simulink model "sim_pos_dist_obs_tcas"  (R2020a)
settings: Solver=ode4  StartTime=0.0  StopTime=30.0  FixedStep=0.01  RelTol=1e-3
values from neighbouring files (symbols this model uses):
  alfa_theta = 20    [draw_compare_dist_pos_obs.m]
  alfa_theta_obs = 100    [draw_compare_dist_pos_obs.m]
  beta1 = 1.2    [draw_compare_dist_pos_obs.m]
  beta2 = 0.8    [draw_compare_dist_pos_obs.m]
  delta_p_i_0 = zeros(3, NF)    [draw_compare_dist_pos_obs.m]
  delta_v_i_0 = zeros(3, NF)    [draw_compare_dist_pos_obs.m]
  dp_aa_t = 0.2 * ones(3, 5) + ( 1.0 - 0.2 ) * rand(3, 5)    [draw_compare_dist_pos_obs.m]
  dp_ff_t = [ 0.4 * ones(1, 5) + ( 1.0 - 0.4 ) * rand(1, 5);                      0.4 * ones(1, 5) + ( 1.0 - 0.4 ) * rand(1, 5);                      0.2 * ones(1, 5) + ( 0.6 - 0.2 ) * rand(1, 5) ]    [draw_compare_dist_pos_obs.m]
  dp_phi_t = ( - pi / 2 ) * ones(3, 5) + ( pi / 2 - ( - pi / 2 ) ) * rand(3, 5)    [draw_compare_dist_pos_obs.m]
  ell1 = [100; 100; 100]    [draw_compare_dist_pos_obs.m]
  ell2 = [50; 50; 50]    [draw_compare_dist_pos_obs.m]
  ell3 = [5; 5; 5]    [draw_compare_dist_pos_obs.m]
  epv = [0.1; 0.1; 0.1]    [draw_compare_dist_pos_obs.m]
  etai_0 = zeros(3,5)    [draw_compare_dist_pos_obs.m]
  k0 = [10; 10; 10]    [draw_compare_dist_pos_obs.m]
  k1v = [0.1; 0.1; 0.1]    [draw_compare_dist_pos_obs.m]
  k2v = [0.1; 0.1; 0.1]    [draw_compare_dist_pos_obs.m]
  k3v = [0.01; 0.01; 0.01]    [draw_compare_dist_pos_obs.m]
  kai_1_t = 0.02    [draw_compare_dist_pos_obs.m]
  kai_3_t = 0.1    [draw_compare_dist_pos_obs.m]
  kai_chi_1 = diag([6; 6; 6])    [draw_compare_dist_pos_obs.m]
  kai_chi_2 = diag([6; 6; 6])    [draw_compare_dist_pos_obs.m]
  kai_u_1 = diag([8; 8; 8])    [draw_compare_dist_pos_obs.m]
  kai_u_2 = diag([8; 8; 8])    [draw_compare_dist_pos_obs.m]
  ksii_0 = zeros(3,5)    [draw_compare_dist_pos_obs.m]
  l1v = diag([20; 20; 20])    [draw_compare_dist_pos_obs.m]
  l2v = diag([30; 30; 30])    [draw_compare_dist_pos_obs.m]
  mass_i = zeros(1,NF)    [draw_compare_dist_pos_obs.m]
  Mii = diag([1;0;0;0;1])    [draw_compare_dist_pos_obs.m]
  pos0 = zeros(3, 1)    [draw_compare_dist_pos_obs.m]
  PZ0 = P0(3)    [draw_compare_dist_pos_obs.m]
  PZ1 = 10    [draw_compare_dist_pos_obs.m]
  Qci_init = repmat([1;0;0;0],1,NF)    [draw_compare_dist_pos_obs.m]
  R0 = 4    [draw_compare_dist_pos_obs.m]
  R1 = 8    [draw_compare_dist_pos_obs.m]
  Rx2 = 10    [draw_compare_dist_pos_obs.m]
  Ry2 = 6    [draw_compare_dist_pos_obs.m]
  Rz2 = 4    [draw_compare_dist_pos_obs.m]
  T0 = 0    [draw_compare_dist_pos_obs.m]
  T1 = tseq1    (= 10)    [draw_compare_dist_pos_obs.m]
  T12 = tseq1 + tseq12    (= 20)    [draw_compare_dist_pos_obs.m]
  T2 = tseq1 + tseq12 + tseq2    (= 30)    [draw_compare_dist_pos_obs.m]
  theta0 = ( 2 / 5 ) * pi    (= 1.25663706144)    [draw_compare_dist_pos_obs.m]
  vel0 = zeros(3, 1)    [draw_compare_dist_pos_obs.m]
  Wij = [0,0,1,0,0;              0,0,1,1,0;              1,0,0,0,1;              0,1,1,0,0;              0,0,1,0,0]    [draw_compare_dist_pos_obs.m]
  X1 = 8    [draw_compare_dist_pos_obs.m]
  X2 = 2    [draw_compare_dist_pos_obs.m]
  X3 = 3    [draw_compare_dist_pos_obs.m]
  Y1 = 10    [draw_compare_dist_pos_obs.m]
  Y2 = 2    [draw_compare_dist_pos_obs.m]
  Y3 = 4    [draw_compare_dist_pos_obs.m]
  Z1 = 4    [draw_compare_dist_pos_obs.m]
  Z2 = -6    [draw_compare_dist_pos_obs.m]
  Z3 = 2    [draw_compare_dist_pos_obs.m]
undefined symbols (not defined in the file or in its folder): cal_frac_squ, p_alfa_1, p_alfa_2, p_beta1, p_beta2, p_dbeta1, p_dbeta2, p_gamma1_pos, p_gamma1_vel, p_gamma2_pos, p_gamma2_vel, q_alfa_1, q_alfa_2, q_beta1, q_beta2, q_dbeta1, q_dbeta2, q_gamma1_pos, q_gamma1_vel, q_gamma2_pos, q_gamma2_vel
(part 2 of 4)

== matlab function sim_pos_dist_obs_tcas/choose ksi_est_err 19 ==
  data: x input; y output
function y = fcn(x)
iiuav = 5;
y = x(:,iiuav);

== matlab function sim_pos_dist_obs_tcas/leader control input ==
  data: t input; u0 output; T1 input; T2 input; R0 input; R1 input; Rx2 input; Ry2 input; Rz2 input
function u0  = fcn(t, T1, T2, R0, R1, Rx2, Ry2, Rz2)
%%%% 给出领导者参考加速度控制输入
u0 = zeros(3, 1);

if t <= ( T1 + 1e-05 )
    u0(1, 1) = - ( 4 * pi * sin( ( 2 * pi * ( t - 0 ) ) / ( 0 - T1 ) ) * ( R0 - R1 ) ) / ( ( 0 - T1 ) ^ 2 ) ...
                        - ( 4 * ( pi ^ 2 ) * cos( ( 2 * pi * ( t - 0 ) ) / ( 0 - T1 ) ) ...
                        * ( R0 + ( ( R0 - R1 ) * ( t - 0 ) ) / ( 0 - T1 ) ) ) / ( ( 0 - T1 ) ^ 2 );
    u0(2, 1) = ( 4 * pi * cos( ( 2 * pi * ( t - 0 ) ) / ( 0 - T1 ) ) * ( R0 - R1 ) ) / ( ( 0 - T1 ) ^ 2 ) ...
                        - ( 4 * ( pi ^ 2 ) * sin( ( 2 * pi * ( t - 0 ) ) / ( 0 - T1 ) ) ...
                        * ( R0 + ( ( R0 - R1 ) * ( t - 0 ) ) / ( 0 - T1 ) ) ) / ( ( 0 - T1 ) ^ 2 );
    u0(3, 1) = 0;
else
    u0(1, 1) = ( 4 * Rx2 * ( pi ^ 2 ) * cos( ( 2 * pi * ( t - T1 ) ) / ( T1 - T2 ) ) ) / ( ( T1 - T2 ) ^ 2 );
    u0(2, 1) = - ( 16 * Ry2 * ( pi ^ 2 ) * sin( ( 4 * pi * ( t - T1 ) ) / ( T1 - T2 ) ) ) / ( ( T1 - T2 ) ^ 2 );
    u0(3, 1) = ( 16 * Rz2 * ( pi ^ 2 ) * sin( ( 4 * pi * ( t - T1 ) ) / ( T1 - T2 ) ) ) / ( ( T1 - T2 ) ^ 2 );
end

== matlab function sim_pos_dist_obs_tcas/choose ksi_est_err 20 ==
  data: x input; y output
function y = fcn(x)
iiuav = 5;
y = x(:,iiuav);

== matlab function sim_pos_dist_obs_tcas/trans to column18 ==
  data: x input; y output
function y = fcn(x)
y = x(:);

== matlab function sim_pos_dist_obs_tcas/trans to column19 ==
  data: x input; y output
function y = fcn(x)
y = x(:);

== matlab function sim_pos_dist_obs_tcas/cal dchi agent 1 ==
  data: kai_chi_1 input; d_chi_1 output; kai_chi_2 input; d_theta_err_ksi_1_vec input; d_theta_err_ksi_2_vec input
function d_chi_1 = fcn(kai_chi_1, kai_chi_2, d_theta_err_ksi_1_vec, d_theta_err_ksi_2_vec)
%%%% 固定时间虚拟速度控制量导数d_chi
iiuav = 1;
d_chi_1 = -kai_chi_1 * d_theta_err_ksi_1_vec(:,iiuav) - kai_chi_2 * d_theta_err_ksi_2_vec(:,iiuav);

== matlab function sim_pos_dist_obs_tcas/combine dtheta_err_ksi ==
  data: d_theta_err_ksi_1_1 input; d_theta_err_ksi_1_2 input; d_theta_err_ksi_1_3 input; d_theta_err_ksi_1_4 input; d_theta_err_ksi_1_5 input; d_theta_err_ksi_1_vec output; d_theta_err_ksi_2_1 input; d_theta_err_ksi_2_vec output; d_theta_err_ksi_2_2 input; d_theta_err_ksi_2_3 input; d_theta_err_ksi_2_4 input; d_theta_err_ksi_2_5 input
function [d_theta_err_ksi_1_vec, d_theta_err_ksi_2_vec]  = fcn(d_theta_err_ksi_1_1, d_theta_err_ksi_1_2, d_theta_err_ksi_1_3, d_theta_err_ksi_1_4, d_theta_err_ksi_1_5, ...
                                                                                                                d_theta_err_ksi_2_1, d_theta_err_ksi_2_2, d_theta_err_ksi_2_3, d_theta_err_ksi_2_4, d_theta_err_ksi_2_5)
%%%% 合并平滑函数的导数
d_theta_err_ksi_1_vec = [d_theta_err_ksi_1_1(:), d_theta_err_ksi_1_2(:), d_theta_err_ksi_1_3(:), d_theta_err_ksi_1_4(:), d_theta_err_ksi_1_5(:)];
d_theta_err_ksi_2_vec = [d_theta_err_ksi_2_1(:), d_theta_err_ksi_2_2(:), d_theta_err_ksi_2_3(:), d_theta_err_ksi_2_4(:), d_theta_err_ksi_2_5(:)];

== matlab function sim_pos_dist_obs_tcas/cal dchi agent 2 ==
  data: kai_chi_1 input; d_chi_2 output; kai_chi_2 input; d_theta_err_ksi_1_vec input; d_theta_err_ksi_2_vec input
function d_chi_2 = fcn(kai_chi_1, kai_chi_2, d_theta_err_ksi_1_vec, d_theta_err_ksi_2_vec)
%%%% 固定时间虚拟速度控制量导数d_chi
iiuav = 2;
d_chi_2 = -kai_chi_1 * d_theta_err_ksi_1_vec(:,iiuav) - kai_chi_2 * d_theta_err_ksi_2_vec(:,iiuav);

== matlab function sim_pos_dist_obs_tcas/cal dchi agent 3 ==
  data: kai_chi_1 input; d_chi_3 output; kai_chi_2 input; d_theta_err_ksi_1_vec input; d_theta_err_ksi_2_vec input
function d_chi_3 = fcn(kai_chi_1, kai_chi_2, d_theta_err_ksi_1_vec, d_theta_err_ksi_2_vec)
%%%% 固定时间虚拟速度控制量导数d_chi
iiuav = 3;
d_chi_3 = -kai_chi_1 * d_theta_err_ksi_1_vec(:,iiuav) - kai_chi_2 * d_theta_err_ksi_2_vec(:,iiuav);

== matlab function sim_pos_dist_obs_tcas/cal dchi agent 4 ==
  data: kai_chi_1 input; d_chi_4 output; kai_chi_2 input; d_theta_err_ksi_1_vec input; d_theta_err_ksi_2_vec input
function d_chi_4 = fcn(kai_chi_1, kai_chi_2, d_theta_err_ksi_1_vec, d_theta_err_ksi_2_vec)
%%%% 固定时间虚拟速度控制量导数d_chi
iiuav = 4;
d_chi_4 = -kai_chi_1 * d_theta_err_ksi_1_vec(:,iiuav) - kai_chi_2 * d_theta_err_ksi_2_vec(:,iiuav);

== matlab function sim_pos_dist_obs_tcas/cal dchi agent 5 ==
  data: kai_chi_1 input; d_chi_5 output; kai_chi_2 input; d_theta_err_ksi_1_vec input; d_theta_err_ksi_2_vec input
function d_chi_5 = fcn(kai_chi_1, kai_chi_2, d_theta_err_ksi_1_vec, d_theta_err_ksi_2_vec)
%%%% 固定时间虚拟速度控制量导数d_chi
iiuav = 5;
d_chi_5 = -kai_chi_1 * d_theta_err_ksi_1_vec(:,iiuav) - kai_chi_2 * d_theta_err_ksi_2_vec(:,iiuav);

== matlab function sim_pos_dist_obs_tcas/combine dchi ==
  data: d_chi_1 input; d_chi_2 input; d_chi_3 input; d_chi_4 input; d_chi_5 input; d_chi_vec output
function d_chi_vec  = fcn(d_chi_1, d_chi_2, d_chi_3, d_chi_4, d_chi_5)
%%%% 合并领导者位置观测器输出结果
d_chi_vec = [d_chi_1(:), d_chi_2(:), d_chi_3(:), d_chi_4(:), d_chi_5(:)];

== matlab function sim_pos_dist_obs_tcas/cal abs 22 ==
  data: x input; y output
function y = fcn(x)
y = abs(x(:));

== matlab function sim_pos_dist_obs_tcas/choose ksi_est_err 21 ==
  data: x input; y output
function y = fcn(x)
iiuav = 1;
y = x(:,iiuav);

== matlab function sim_pos_dist_obs_tcas/cal x1_tilt ==
  data: ksi_i_vec input; x1_hat_vec input; x1_tilt_vec output
function x1_tilt_vec = fcn(ksi_i_vec, x1_hat_vec)
%%%% 计算状态观测误差
x1_tilt_vec = zeros(3,5);
for iiuav = 1:5
    x1_tilt_vec(:,iiuav) = ksi_i_vec(:,iiuav) - x1_hat_vec(:,iiuav);
end

== matlab function sim_pos_dist_obs_tcas/cal err_1_x1_tilt ==
  data: ell1 input; epv input; err_1_x1_tilt_vec output; x1_tilt_vec input
function err_1_x1_tilt_vec = fcn(ell1, epv, x1_tilt_vec)
%%%% 计算状态观测误差
err_1_x1_tilt_vec = zeros(3,5);
for iiuav = 1:5
    err_1_x1_tilt_vec(:,iiuav) = (1 ./ (ell1(:) .* (epv(:) .^ 2))) .* x1_tilt_vec(:,iiuav);
end

== matlab function sim_pos_dist_obs_tcas/cal err_2_x1_tilt ==
  data: ell2 input; epv input; err_2_x1_tilt_vec output; x1_tilt_vec input
function err_2_x1_tilt_vec = fcn(ell2, epv, x1_tilt_vec)
%%%% 计算状态观测误差
err_2_x1_tilt_vec = zeros(3,5);
for iiuav = 1:5
    err_2_x1_tilt_vec(:,iiuav) = (1 ./ (ell2(:) .* (epv(:) .^ 2))) .* x1_tilt_vec(:,iiuav);
end

== matlab function sim_pos_dist_obs_tcas/generate translational disturbance agent 5 ==
  data: dp_aa_t input; dp_ff_t input; dp_phi_t input; dp_5 output; t input
function dp_5 = fcn(dp_aa_t, dp_ff_t, dp_phi_t, t)
%%%% 平移动力学方程中的扰动项设置
epsil_t = zeros(3, 1);

for kk = 1:5
    epsil_t = epsil_t + dp_aa_t(:, kk) .* sin( 2 * pi * dp_ff_t(:, kk) * t + dp_phi_t(:, kk) );
end

dp_5 = [ epsil_t(1) + 1.6 * sin( 0.2 * t ) + 2.0 * cos( 0.3 * t ) + 1.4 * sin( 0.5 * t ) ...
                + 4 * exp( -0.1 * t ) * sin( 0.5 * t ) + 3 / ( 1 + exp( -0.2 * ( t - 15 ) ) ); ...
                epsil_t(2) + 1.2 * sin( 0.1 * t ) + 3 * cos( 0.2 * t ) + 0.8 * sin( 0.4 * t ) ...
                + 2 * exp( -0.15 * t ) * cos( 0.6 * t ) + 3 / ( 1 + exp( -0.3 * ( t - 25 ) ) ); ...
                epsil_t(3) + 1.8 * sin( 0.1 * t ) + 1.6 * sin( 0.2 * t ) + 1.6 * cos( 0.3 * t ) ...
                + 4 * exp( -0.05 * t ) * sin( 0.4 * t + pi / 4 ) + 3 / ( 1 + exp( -0.5 * ( t - 20 ) ) ) ];

== matlab function sim_pos_dist_obs_tcas/cal err_3_x1_tilt ==
  data: ell3 input; epv input; err_3_x1_tilt_vec output; x1_tilt_vec input
function err_3_x1_tilt_vec = fcn(ell3, epv, x1_tilt_vec)
%%%% 计算状态观测误差
err_3_x1_tilt_vec = zeros(3,5);
for iiuav = 1:5
    err_3_x1_tilt_vec(:,iiuav) = (ell3(:) ./ (epv(:) .^ 2)) .* x1_tilt_vec(:,iiuav);
end

== matlab function sim_pos_dist_obs_tcas/cal abs 23 ==
  data: x input; y output
function y = fcn(x)
y = abs(x(:));

== matlab function sim_pos_dist_obs_tcas/cal abs 24 ==
  data: x input; y output
function y = fcn(x)
y = abs(x(:));

== matlab function sim_pos_dist_obs_tcas/choose ksi_est_err 22 ==
  data: x input; y output
function y = fcn(x)
iiuav = 1;
y = x(:,iiuav);

== matlab function sim_pos_dist_obs_tcas/choose ksi_est_err 23 ==
  data: x input; y output
function y = fcn(x)
iiuav = 1;
y = x(:,iiuav);

== matlab function sim_pos_dist_obs_tcas/choose ksi_est_err 24 ==
  data: x input; y output
function y = fcn(x)
iiuav = 1;
y = x(:,iiuav);

== matlab function sim_pos_dist_obs_tcas/trans to column20 ==
  data: x input; y output
function y = fcn(x)
y = x(:);

== matlab function sim_pos_dist_obs_tcas/cal abs 25 ==
  data: x input; y output
function y = fcn(x)
y = abs(x(:));

== matlab function sim_pos_dist_obs_tcas/cal abs 26 ==
  data: x input; y output
function y = fcn(x)
y = abs(x(:));

== matlab function sim_pos_dist_obs_tcas/choose ksi_est_err 25 ==
  data: x input; y output
function y = fcn(x)
iiuav = 1;
y = x(:,iiuav);

== matlab function sim_pos_dist_obs_tcas/choose ksi_est_err 26 ==
  data: x input; y output
function y = fcn(x)
iiuav = 1;
y = x(:,iiuav);

== matlab function sim_pos_dist_obs_tcas/trans to column21 ==
  data: x input; y output
function y = fcn(x)
y = x(:);

== matlab function sim_pos_dist_obs_tcas/trans to column22 ==
  data: x input; y output
function y = fcn(x)
y = x(:);

== matlab function sim_pos_dist_obs_tcas/cal G_fun_x1_tilt agent 2 ==
  data: err_1_x1_tilt_vec input; err_2_x1_tilt_vec input; G_fun_x1_tilt_1_2 output; err_3_x1_tilt_vec input; err_x1_alfa_squ_1_2 input; G_fun_x1_tilt_2_2 output; err_x1_alfa_squ_2_2 input; err_x1_alfa_squ_3_2 input; err_x1_alfa_squ_4_2 input; err_x1_alfa_squ_5_2 input; err_x1_alfa_squ_6_2 input; G_fun_x1_tilt_3_2 output
function [G_fun_x1_tilt_1_2, G_fun_x1_tilt_2_2, G_fun_x1_tilt_3_2] = fcn(err_1_x1_tilt_vec, err_2_x1_tilt_vec, err_3_x1_tilt_vec, ...
                                                                                                                                err_x1_alfa_squ_1_2, err_x1_alfa_squ_2_2, err_x1_alfa_squ_3_2, ...
                                                                                                                                err_x1_alfa_squ_4_2, err_x1_alfa_squ_5_2, err_x1_alfa_squ_6_2)
%%%% 计算平滑递增函数
iiuav = 2;
G_fun_x1_tilt_1_2 = tanh(err_x1_alfa_squ_2_2(:)) .* err_x1_alfa_squ_1_2(:) .* sign(err_1_x1_tilt_vec(:,iiuav));
G_fun_x1_tilt_2_2 = tanh(err_x1_alfa_squ_4_2(:)) .* err_x1_alfa_squ_3_2(:) .* sign(err_2_x1_tilt_vec(:,iiuav));
G_fun_x1_tilt_3_2 = tanh(err_x1_alfa_squ_6_2(:)) .* err_x1_alfa_squ_5_2(:) .* sign(err_3_x1_tilt_vec(:,iiuav));

== matlab function sim_pos_dist_obs_tcas/combine translational disturbance ==
  data: dp_vec output; dp_1 input; dp_2 input; dp_3 input; dp_4 input; dp_5 input
function dp_vec = fcn(dp_1, dp_2, dp_3, dp_4, dp_5)
%%%% 合并领导者编队跟踪误差结果
dp_vec = [dp_1(:), dp_2(:), dp_3(:), dp_4(:), dp_5(:)];

== matlab function sim_pos_dist_obs_tcas/cal abs 27 ==
  data: x input; y output
function y = fcn(x)
y = abs(x(:));

== matlab function sim_pos_dist_obs_tcas/cal abs 28 ==
  data: x input; y output
function y = fcn(x)
y = abs(x(:));

== matlab function sim_pos_dist_obs_tcas/cal abs 29 ==
  data: x input; y output
function y = fcn(x)
y = abs(x(:));

== matlab function sim_pos_dist_obs_tcas/cal Rei ==
  data: Rei output; Qei input
function Rei = fcn(Qei)
%%%% 使用罗德里格公式由四元数Qei求解Rei
Rei = zeros(3,3,5);
for iuav = 1:5
    thetaei_tmp = Qei(1,iuav);
    qei_tmp = Qei(2:4,iuav);
    Rei(:,:,iuav) = ((thetaei_tmp^2) - (qei_tmp')*qei_tmp) * eye(3,3) ...
                            + 2 * qei_tmp * (qei_tmp') ...
                            - 2 * thetaei_tmp * cal_askew_mat(qei_tmp);
end

end

== matlab function sim_pos_dist_obs_tcas/cal abs 30 ==
  data: x input; y output
function y = fcn(x)
y = abs(x(:));

== matlab function sim_pos_dist_obs_tcas/cal abs 61 ==
  data: x input; y output
function y = fcn(x)
y = abs(x(:));

== matlab function sim_pos_dist_obs_tcas/cal abs 62 ==
  data: x input; y output
function y = fcn(x)
y = abs(x(:));

== matlab function sim_pos_dist_obs_tcas/choose ksi_est_err 27 ==
  data: x input; y output
function y = fcn(x)
iiuav = 2;
y = x(:,iiuav);

== matlab function sim_pos_dist_obs_tcas/choose ksi_est_err 28 ==
  data: x input; y output
function y = fcn(x)
iiuav = 2;
y = x(:,iiuav);

== matlab function sim_pos_dist_obs_tcas/choose ksi_est_err 29 ==
  data: x input; y output
function y = fcn(x)
iiuav = 2;
y = x(:,iiuav);

== matlab function sim_pos_dist_obs_tcas/choose ksi_est_err 30 ==
  data: x input; y output
function y = fcn(x)
iiuav = 2;
y = x(:,iiuav);

== matlab function sim_pos_dist_obs_tcas/choose ksi_est_err 41 ==
  data: x input; y output
function y = fcn(x)
iiuav = 2;
y = x(:,iiuav);

== matlab function sim_pos_dist_obs_tcas/choose ksi_est_err 42 ==
  data: x input; y output
function y = fcn(x)
iiuav = 2;
y = x(:,iiuav);

== matlab function sim_pos_dist_obs_tcas/trans to column23 ==
  data: x input; y output
function y = fcn(x)
y = x(:);

== matlab function sim_pos_dist_obs_tcas/cal abs 2 ==
  data: x input; y output
function y = fcn(x)
y = abs(x(:));

== matlab function sim_pos_dist_obs_tcas/trans to column24 ==
  data: x input; y output
function y = fcn(x)
y = x(:);

== matlab function sim_pos_dist_obs_tcas/trans to column25 ==
  data: x input; y output
function y = fcn(x)
y = x(:);

== matlab function sim_pos_dist_obs_tcas/trans to column26 ==
  data: x input; y output
function y = fcn(x)
y = x(:);

== matlab function sim_pos_dist_obs_tcas/trans to column27 ==
  data: x input; y output
function y = fcn(x)
y = x(:);

== matlab function sim_pos_dist_obs_tcas/trans to column28 ==
  data: x input; y output
function y = fcn(x)
y = x(:);

== matlab function sim_pos_dist_obs_tcas/depart Re5 ==
  data: y output; x input
function y = fcn(x)
y = x(:,:,5);

end

== matlab function sim_pos_dist_obs_tcas/depart Re1 ==
  data: y output; x input
function y = fcn(x)
y = x(:,:,1);

end

== matlab function sim_pos_dist_obs_tcas/depart Re2 ==
  data: y output; x input
function y = fcn(x)
y = x(:,:,2);

end

== matlab function sim_pos_dist_obs_tcas/depart Re3 ==
  data: y output; x input
function y = fcn(x)
y = x(:,:,3);

end

== matlab function sim_pos_dist_obs_tcas/depart Re4 ==
  data: y output; x input
function y = fcn(x)
y = x(:,:,4);

end

== matlab function sim_pos_dist_obs_tcas/cal theta_err_ksi agent 1 ==
  data: alfa_theta input; err_ksi_squ_1_node_1 input; theta_err_ksi_1_1 output; err_ksi_squ_2_node_1 input; err_ksi_vec input; theta_err_ksi_2_1 output
function [theta_err_ksi_1_1, theta_err_ksi_2_1] = fcn(alfa_theta, err_ksi_squ_1_node_1, err_ksi_squ_2_node_1, err_ksi_vec)
%%%% 计算平滑递增函数
iiuav = 1;
theta_err_ksi_1_1 = err_ksi_squ_1_node_1(:) .* ( -1 + 2 ./ ( 1 + exp( -alfa_theta .* err_ksi_vec(:,iiuav) ) ) );
theta_err_ksi_2_1 = err_ksi_squ_2_node_1(:) .* ( -1 + 2 ./ ( 1 + exp( -alfa_theta .* err_ksi_vec(:,iiuav) ) ) );

== matlab function sim_pos_dist_obs_tcas/cal G_fun_x1_tilt agent 3 ==
  data: err_1_x1_tilt_vec input; err_2_x1_tilt_vec input; G_fun_x1_tilt_1_3 output; err_3_x1_tilt_vec input; err_x1_alfa_squ_1_3 input; G_fun_x1_tilt_2_3 output; err_x1_alfa_squ_2_3 input; err_x1_alfa_squ_3_3 input; err_x1_alfa_squ_4_3 input; err_x1_alfa_squ_5_3 input; err_x1_alfa_squ_6_3 input; G_fun_x1_tilt_3_3 output
function [G_fun_x1_tilt_1_3, G_fun_x1_tilt_2_3, G_fun_x1_tilt_3_3] = fcn(err_1_x1_tilt_vec, err_2_x1_tilt_vec, err_3_x1_tilt_vec, ...
                                                                                                                                err_x1_alfa_squ_1_3, err_x1_alfa_squ_2_3, err_x1_alfa_squ_3_3, ...
                                                                                                                                err_x1_alfa_squ_4_3, err_x1_alfa_squ_5_3, err_x1_alfa_squ_6_3)
%%%% 计算平滑递增函数
iiuav = 3;
G_fun_x1_tilt_1_3 = tanh(err_x1_alfa_squ_2_3(:)) .* err_x1_alfa_squ_1_3(:) .* sign(err_1_x1_tilt_vec(:,iiuav));
G_fun_x1_tilt_2_3 = tanh(err_x1_alfa_squ_4_3(:)) .* err_x1_alfa_squ_3_3(:) .* sign(err_2_x1_tilt_vec(:,iiuav));
G_fun_x1_tilt_3_3 = tanh(err_x1_alfa_squ_6_3(:)) .* err_x1_alfa_squ_5_3(:) .* sign(err_3_x1_tilt_vec(:,iiuav));

== matlab function sim_pos_dist_obs_tcas/cal abs 63 ==
  data: x input; y output
function y = fcn(x)
y = abs(x(:));

== matlab function sim_pos_dist_obs_tcas/cal abs 64 ==
  data: x input; y output
function y = fcn(x)
y = abs(x(:));

== matlab function sim_pos_dist_obs_tcas/cal abs 65 ==
  data: x input; y output
function y = fcn(x)
y = abs(x(:));

== matlab function sim_pos_dist_obs_tcas/cal abs 66 ==
  data: x input; y output
function y = fcn(x)
y = abs(x(:));

== matlab function sim_pos_dist_obs_tcas/choose ksi_est_err 1 ==
  data: x input; y output
function y = fcn(x)
iiuav = 1;
y = x(:,iiuav);

== matlab function sim_pos_dist_obs_tcas/trans to column35 ==
  data: x input; y output
function y = fcn(x)
y = x(:);

== matlab function sim_pos_dist_obs_tcas/cal abs 67 ==
  data: x input; y output
function y = fcn(x)
y = abs(x(:));

== matlab function sim_pos_dist_obs_tcas/cal abs 68 ==
  data: x input; y output
function y = fcn(x)
y = abs(x(:));

== matlab function sim_pos_dist_obs_tcas/choose ksi_est_err 43 ==
  data: x input; y output
function y = fcn(x)
iiuav = 3;
y = x(:,iiuav);

== matlab function sim_pos_dist_obs_tcas/choose ksi_est_err 44 ==
  data: x input; y output
function y = fcn(x)
iiuav = 3;
y = x(:,iiuav);

== matlab function sim_pos_dist_obs_tcas/choose ksi_est_err 45 ==
  data: x input; y output
function y = fcn(x)
iiuav = 3;
y = x(:,iiuav);

== matlab function sim_pos_dist_obs_tcas/choose ksi_est_err 46 ==
  data: x input; y output
function y = fcn(x)
iiuav = 3;
y = x(:,iiuav);

== matlab function sim_pos_dist_obs_tcas/choose ksi_est_err 47 ==
  data: x input; y output
function y = fcn(x)
iiuav = 3;
y = x(:,iiuav);

== matlab function sim_pos_dist_obs_tcas/choose ksi_est_err 48 ==
  data: x input; y output
function y = fcn(x)
iiuav = 3;
y = x(:,iiuav);

== matlab function sim_pos_dist_obs_tcas/trans to column1 ==
  data: x input; y output
function y = fcn(x)
y = x(:);

== matlab function sim_pos_dist_obs_tcas/trans to column29 ==
  data: x input; y output
function y = fcn(x)
y = x(:);

== matlab function sim_pos_dist_obs_tcas/trans to column61 ==
  data: x input; y output
function y = fcn(x)
y = x(:);

== matlab function sim_pos_dist_obs_tcas/trans to column62 ==
  data: x input; y output
function y = fcn(x)
y = x(:);

== matlab function sim_pos_dist_obs_tcas/trans to column63 ==
  data: x input; y output
function y = fcn(x)
y = x(:);

== matlab function sim_pos_dist_obs_tcas/trans to column64 ==
  data: x input; y output
function y = fcn(x)
y = x(:);

== matlab function sim_pos_dist_obs_tcas/trans to column65 ==
  data: x input; y output
function y = fcn(x)
y = x(:);

== matlab function sim_pos_dist_obs_tcas/cal G_fun_x1_tilt agent 4 ==
  data: err_1_x1_tilt_vec input; err_2_x1_tilt_vec input; G_fun_x1_tilt_1_4 output; err_3_x1_tilt_vec input; err_x1_alfa_squ_1_4 input; G_fun_x1_tilt_2_4 output; err_x1_alfa_squ_2_4 input; err_x1_alfa_squ_3_4 input; err_x1_alfa_squ_4_4 input; err_x1_alfa_squ_5_4 input; err_x1_alfa_squ_6_4 input; G_fun_x1_tilt_3_4 output
function [G_fun_x1_tilt_1_4, G_fun_x1_tilt_2_4, G_fun_x1_tilt_3_4] = fcn(err_1_x1_tilt_vec, err_2_x1_tilt_vec, err_3_x1_tilt_vec, ...
                                                                                                                                err_x1_alfa_squ_1_4, err_x1_alfa_squ_2_4, err_x1_alfa_squ_3_4, ...
                                                                                                                                err_x1_alfa_squ_4_4, err_x1_alfa_squ_5_4, err_x1_alfa_squ_6_4)
%%%% 计算平滑递增函数
iiuav = 4;
G_fun_x1_tilt_1_4 = tanh(err_x1_alfa_squ_2_4(:)) .* err_x1_alfa_squ_1_4(:) .* sign(err_1_x1_tilt_vec(:,iiuav));
G_fun_x1_tilt_2_4 = tanh(err_x1_alfa_squ_4_4(:)) .* err_x1_alfa_squ_3_4(:) .* sign(err_2_x1_tilt_vec(:,iiuav));
G_fun_x1_tilt_3_4 = tanh(err_x1_alfa_squ_6_4(:)) .* err_x1_alfa_squ_5_4(:) .* sign(err_3_x1_tilt_vec(:,iiuav));

== matlab function sim_pos_dist_obs_tcas/cal abs 69 ==
  data: x input; y output
function y = fcn(x)
y = abs(x(:));

== matlab function sim_pos_dist_obs_tcas/cal abs 3 ==
  data: x input; y output
function y = fcn(x)
y = abs(x(:));

== matlab function sim_pos_dist_obs_tcas/cal abs 70 ==
  data: x input; y output
function y = fcn(x)
y = abs(x(:));

== matlab function sim_pos_dist_obs_tcas/cal abs 71 ==
  data: x input; y output
function y = fcn(x)
y = abs(x(:));

== matlab function sim_pos_dist_obs_tcas/cal abs 72 ==
  data: x input; y output
function y = fcn(x)
y = abs(x(:));

== matlab function sim_pos_dist_obs_tcas/cal Rci from ui ==
  data: Rci output; mi input; ui input
function Rci = fcn(mi, ui)
Rci = zeros(3,3,5);
for iiuav = 1:5
    Rci(:,:,iiuav) = cal_Rc_with_u(mi(iiuav), ui(:,iiuav));
end

end

== matlab function sim_pos_dist_obs_tcas/cal abs 73 ==
  data: x input; y output
function y = fcn(x)
y = abs(x(:));

== matlab function sim_pos_dist_obs_tcas/cal abs 74 ==
  data: x input; y output
function y = fcn(x)
y = abs(x(:));

== matlab function sim_pos_dist_obs_tcas/choose ksi_est_err 49 ==
  data: x input; y output
function y = fcn(x)
iiuav = 4;
y = x(:,iiuav);

== matlab function sim_pos_dist_obs_tcas/choose ksi_est_err 50 ==
  data: x input; y output
function y = fcn(x)
iiuav = 4;
y = x(:,iiuav);

== matlab function sim_pos_dist_obs_tcas/choose ksi_est_err 51 ==
  data: x input; y output
function y = fcn(x)
iiuav = 4;
y = x(:,iiuav);

== matlab function sim_pos_dist_obs_tcas/choose ksi_est_err 52 ==
  data: x input; y output
function y = fcn(x)
iiuav = 4;
y = x(:,iiuav);

== matlab function sim_pos_dist_obs_tcas/cal abs 4 ==
  data: x input; y output
function y = fcn(x)
y = abs(x(:));

== matlab function sim_pos_dist_obs_tcas/choose ksi_est_err 53 ==
  data: x input; y output
function y = fcn(x)
iiuav = 4;
y = x(:,iiuav);

== matlab function sim_pos_dist_obs_tcas/choose ksi_est_err 54 ==
  data: x input; y output
function y = fcn(x)
iiuav = 4;
y = x(:,iiuav);

== matlab function sim_pos_dist_obs_tcas/trans to column66 ==
  data: x input; y output
function y = fcn(x)
y = x(:);

== matlab function sim_pos_dist_obs_tcas/trans to column67 ==
  data: x input; y output
function y = fcn(x)
y = x(:);

== matlab function sim_pos_dist_obs_tcas/trans to column68 ==
  data: x input; y output
function y = fcn(x)
y = x(:);

== matlab function sim_pos_dist_obs_tcas/trans to column69 ==
  data: x input; y output
function y = fcn(x)
y = x(:);

== matlab function sim_pos_dist_obs_tcas/trans to column70 ==
  data: x input; y output
function y = fcn(x)
y = x(:);

== matlab function sim_pos_dist_obs_tcas/trans to column71 ==
  data: x input; y output
function y = fcn(x)
y = x(:);

== matlab function sim_pos_dist_obs_tcas/cal G_fun_x1_tilt agent 5 ==
  data: err_1_x1_tilt_vec input; err_2_x1_tilt_vec input; G_fun_x1_tilt_1_5 output; err_3_x1_tilt_vec input; err_x1_alfa_squ_1_5 input; G_fun_x1_tilt_2_5 output; err_x1_alfa_squ_2_5 input; err_x1_alfa_squ_3_5 input; err_x1_alfa_squ_4_5 input; err_x1_alfa_squ_5_5 input; err_x1_alfa_squ_6_5 input; G_fun_x1_tilt_3_5 output
function [G_fun_x1_tilt_1_5, G_fun_x1_tilt_2_5, G_fun_x1_tilt_3_5] = fcn(err_1_x1_tilt_vec, err_2_x1_tilt_vec, err_3_x1_tilt_vec, ...
                                                                                                                                err_x1_alfa_squ_1_5, err_x1_alfa_squ_2_5, err_x1_alfa_squ_3_5, ...
                                                                                                                                err_x1_alfa_squ_4_5, err_x1_alfa_squ_5_5, err_x1_alfa_squ_6_5)
%%%% 计算平滑递增函数
iiuav = 5;
G_fun_x1_tilt_1_5 = tanh(err_x1_alfa_squ_2_5(:)) .* err_x1_alfa_squ_1_5(:) .* sign(err_1_x1_tilt_vec(:,iiuav));
G_fun_x1_tilt_2_5 = tanh(err_x1_alfa_squ_4_5(:)) .* err_x1_alfa_squ_3_5(:) .* sign(err_2_x1_tilt_vec(:,iiuav));
G_fun_x1_tilt_3_5 = tanh(err_x1_alfa_squ_6_5(:)) .* err_x1_alfa_squ_5_5(:) .* sign(err_3_x1_tilt_vec(:,iiuav));

== matlab function sim_pos_dist_obs_tcas/cal theta_err_ksi agent 2 ==
  data: alfa_theta input; err_ksi_squ_1_node_2 input; theta_err_ksi_1_2 output; err_ksi_squ_2_node_2 input; err_ksi_vec input; theta_err_ksi_2_2 output
function [theta_err_ksi_1_2, theta_err_ksi_2_2] = fcn(alfa_theta, err_ksi_squ_1_node_2, err_ksi_squ_2_node_2, err_ksi_vec)
%%%% 计算平滑递增函数
iiuav = 2;
theta_err_ksi_1_2 = err_ksi_squ_1_node_2(:) .* ( -1 + 2 ./ ( 1 + exp( -alfa_theta .* err_ksi_vec(:,iiuav) ) ) );
theta_err_ksi_2_2 = err_ksi_squ_2_node_2(:) .* ( -1 + 2 ./ ( 1 + exp( -alfa_theta .* err_ksi_vec(:,iiuav) ) ) );

== matlab function sim_pos_dist_obs_tcas/cal abs 75 ==
  data: x input; y output
function y = fcn(x)
y = abs(x(:));

== matlab function sim_pos_dist_obs_tcas/cal abs 76 ==
  data: x input; y output
function y = fcn(x)
y = abs(x(:));

== matlab function sim_pos_dist_obs_tcas/cal abs 77 ==
  data: x input; y output
function y = fcn(x)
y = abs(x(:));

== matlab function sim_pos_dist_obs_tcas/cal abs 78 ==
  data: x input; y output
function y = fcn(x)
y = abs(x(:));

== matlab function sim_pos_dist_obs_tcas/cal abs 79 ==
  data: x input; y output
function y = fcn(x)
y = abs(x(:));

== matlab function sim_pos_dist_obs_tcas/cal abs 80 ==
  data: x input; y output
function y = fcn(x)
y = abs(x(:));

== matlab function sim_pos_dist_obs_tcas/choose ksi_est_err 55 ==
  data: x input; y output
function y = fcn(x)
iiuav = 5;
y = x(:,iiuav);

== matlab function sim_pos_dist_obs_tcas/choose ksi_est_err 56 ==
  data: x input; y output
function y = fcn(x)
iiuav = 5;
y = x(:,iiuav);

== matlab function sim_pos_dist_obs_tcas/choose ksi_est_err 57 ==
  data: x input; y output
function y = fcn(x)
iiuav = 5;
y = x(:,iiuav);

== matlab function sim_pos_dist_obs_tcas/choose ksi_est_err 58 ==
  data: x input; y output
function y = fcn(x)
iiuav = 5;
y = x(:,iiuav);

== matlab function sim_pos_dist_obs_tcas/choose ksi_est_err 59 ==
  data: x input; y output
function y = fcn(x)
iiuav = 5;
y = x(:,iiuav);

== matlab function sim_pos_dist_obs_tcas/choose ksi_est_err 60 ==
  data: x input; y output
function y = fcn(x)
iiuav = 5;
y = x(:,iiuav);

== matlab function sim_pos_dist_obs_tcas/trans to column72 ==
  data: x input; y output
function y = fcn(x)
y = x(:);

== matlab function sim_pos_dist_obs_tcas/trans to column73 ==
  data: x input; y output
function y = fcn(x)
y = x(:);

== matlab function sim_pos_dist_obs_tcas/trans to column74 ==
  data: x input; y output
function y = fcn(x)
y = x(:);

== matlab function sim_pos_dist_obs_tcas/choose ksi_est_err 3 ==
  data: x input; y output
function y = fcn(x)
iiuav = 2;
y = x(:,iiuav);

== matlab function sim_pos_dist_obs_tcas/trans to column75 ==
  data: x input; y output
function y = fcn(x)
y = x(:);

== matlab function sim_pos_dist_obs_tcas/trans to column76 ==
  data: x input; y output
function y = fcn(x)
y = x(:);

== matlab function sim_pos_dist_obs_tcas/trans to column77 ==
  data: x input; y output
function y = fcn(x)
y = x(:);

== matlab function sim_pos_dist_obs_tcas/combine G_fun_x1_tilt ==
  data: G_fun_x1_tilt_1_1 input; G_fun_x1_tilt_1_2 input; G_fun_x1_tilt_1_vec output; G_fun_x1_tilt_1_3 input; G_fun_x1_tilt_1_4 input; G_fun_x1_tilt_2_vec output; G_fun_x1_tilt_1_5 input; G_fun_x1_tilt_2_1 input; G_fun_x1_tilt_2_2 input; G_fun_x1_tilt_2_3 input; G_fun_x1_tilt_2_4 input; G_fun_x1_tilt_3_vec output; G_fun_x1_tilt_2_5 input; G_fun_x1_tilt_3_1 input; G_fun_x1_tilt_3_2 input; G_fun_x1_tilt_3_3 input; G_fun_x1_tilt_3_4 input; G_fun_x1_tilt_3_5 input
function [G_fun_x1_tilt_1_vec, G_fun_x1_tilt_2_vec, G_fun_x1_tilt_3_vec] = fcn(G_fun_x1_tilt_1_1, G_fun_x1_tilt_1_2, G_fun_x1_tilt_1_3, G_fun_x1_tilt_1_4, G_fun_x1_tilt_1_5, ...
                                                                                                                                            G_fun_x1_tilt_2_1, G_fun_x1_tilt_2_2, G_fun_x1_tilt_2_3, G_fun_x1_tilt_2_4, G_fun_x1_tilt_2_5, ...
                                                                                                                                            G_fun_x1_tilt_3_1, G_fun_x1_tilt_3_2, G_fun_x1_tilt_3_3, G_fun_x1_tilt_3_4, G_fun_x1_tilt_3_5)
G_fun_x1_tilt_1_vec = [G_fun_x1_tilt_1_1(:), G_fun_x1_tilt_1_2(:), G_fun_x1_tilt_1_3(:), G_fun_x1_tilt_1_4(:), G_fun_x1_tilt_1_5];
G_fun_x1_tilt_2_vec = [G_fun_x1_tilt_2_1(:), G_fun_x1_tilt_2_2(:), G_fun_x1_tilt_2_3(:), G_fun_x1_tilt_2_4(:), G_fun_x1_tilt_2_5];
G_fun_x1_tilt_3_vec = [G_fun_x1_tilt_3_1(:), G_fun_x1_tilt_3_2(:), G_fun_x1_tilt_3_3(:), G_fun_x1_tilt_3_4(:), G_fun_x1_tilt_3_5];

== matlab function sim_pos_dist_obs_tcas/cal x1_hat agent 1 ==
  data: k0 input; k1v input; d_x1_hat_1 output; ell1 input; epv input; x2_hat_vec input; x1_tilt_vec input; G_fun_x1_tilt_1_vec input
function d_x1_hat_1 = fcn(k0, k1v, ell1, epv, x2_hat_vec, x1_tilt_vec, G_fun_x1_tilt_1_vec)
%%%% 计算状态观测误差
iiuav = 1;
d_x1_hat_1 = x2_hat_vec(:,iiuav) + k1v(:) .* ( (x1_tilt_vec(:,iiuav) ./ epv(:)) + ...
                                                                epv(:) .* k0(:) .* ell1(:) .* G_fun_x1_tilt_1_vec(:,iiuav) );

== matlab function sim_pos_dist_obs_tcas/cal x1_hat agent 2 ==
  data: k0 input; k1v input; d_x1_hat_2 output; ell1 input; epv input; x2_hat_vec input; x1_tilt_vec input; G_fun_x1_tilt_1_vec input
function d_x1_hat_2 = fcn(k0, k1v, ell1, epv, x2_hat_vec, x1_tilt_vec, G_fun_x1_tilt_1_vec)
%%%% 计算状态观测误差
iiuav = 2;
d_x1_hat_2 = x2_hat_vec(:,iiuav) + k1v(:) .* ( (x1_tilt_vec(:,iiuav) ./ epv(:)) + ...
                                                                epv(:) .* k0(:) .* ell1(:) .* G_fun_x1_tilt_1_vec(:,iiuav) );

== matlab function sim_pos_dist_obs_tcas/choose ksi_est_err 4 ==
  data: x input; y output
function y = fcn(x)
iiuav = 2;
y = x(:,iiuav);

== matlab function sim_pos_dist_obs_tcas/cal x1_hat agent 3 ==
  data: k0 input; k1v input; d_x1_hat_3 output; ell1 input; epv input; x2_hat_vec input; x1_tilt_vec input; G_fun_x1_tilt_1_vec input
function d_x1_hat_3 = fcn(k0, k1v, ell1, epv, x2_hat_vec, x1_tilt_vec, G_fun_x1_tilt_1_vec)
%%%% 计算状态观测误差
iiuav = 3;
d_x1_hat_3 = x2_hat_vec(:,iiuav) + k1v(:) .* ( (x1_tilt_vec(:,iiuav) ./ epv(:)) + ...
                                                                epv(:) .* k0(:) .* ell1(:) .* G_fun_x1_tilt_1_vec(:,iiuav) );

== matlab function sim_pos_dist_obs_tcas/cal x1_hat agent 4 ==
  data: k0 input; k1v input; d_x1_hat_4 output; ell1 input; epv input; x2_hat_vec input; x1_tilt_vec input; G_fun_x1_tilt_1_vec input
function d_x1_hat_4 = fcn(k0, k1v, ell1, epv, x2_hat_vec, x1_tilt_vec, G_fun_x1_tilt_1_vec)
%%%% 计算状态观测误差
iiuav = 4;
d_x1_hat_4 = x2_hat_vec(:,iiuav) + k1v(:) .* ( (x1_tilt_vec(:,iiuav) ./ epv(:)) + ...
                                                                epv(:) .* k0(:) .* ell1(:) .* G_fun_x1_tilt_1_vec(:,iiuav) );

== matlab function sim_pos_dist_obs_tcas/cal x1_hat agent 5 ==
  data: k0 input; k1v input; d_x1_hat_5 output; ell1 input; epv input; x2_hat_vec input; x1_tilt_vec input; G_fun_x1_tilt_1_vec input
function d_x1_hat_5 = fcn(k0, k1v, ell1, epv, x2_hat_vec, x1_tilt_vec, G_fun_x1_tilt_1_vec)
%%%% 计算状态观测误差
iiuav = 5;
d_x1_hat_5 = x2_hat_vec(:,iiuav) + k1v(:) .* ( (x1_tilt_vec(:,iiuav) ./ epv(:)) + ...
                                                                epv(:) .* k0(:) .* ell1(:) .* G_fun_x1_tilt_1_vec(:,iiuav) );

== matlab function sim_pos_dist_obs_tcas/combine x1_hat ==
  data: x1_hat_1 input; x1_hat_2 input; x1_hat_3 input; x1_hat_4 input; x1_hat_5 input; x1_hat_vec output
function x1_hat_vec  = fcn(x1_hat_1, x1_hat_2, x1_hat_3, x1_hat_4, x1_hat_5)
%%%% 合并领导者位置观测器输出结果
x1_hat_vec = [x1_hat_1(:), x1_hat_2(:), x1_hat_3(:), x1_hat_4(:), x1_hat_5(:)];

== matlab function sim_pos_dist_obs_tcas/cal x2_hat agent 1 ==
  data: k0 input; k2v input; d_x2_hat_1 output; ell2 input; epv input; Ri input; ui input; dp_hat_vec input; x1_tilt_vec input; G_fun_x1_tilt_2_vec input
function d_x2_hat_1 = fcn(k0, k2v, ell2, epv, Ri, ui, dp_hat_vec, x1_tilt_vec, G_fun_x1_tilt_2_vec)
%%%% 计算状态观测误差
iiuav = 1;
g0 = 9.80663;
e3 = [0;0;1];
d_x2_hat_1 = dp_hat_vec(:,iiuav) + k2v(:) .* ( (x1_tilt_vec(:,iiuav) ./ (epv(:) .^ 2)) + ...
                                                                (k0(:) .^ 2) .* ell2(:) .* G_fun_x1_tilt_2_vec(:,iiuav) ) + ...
                                                                - g0 * e3 + norm(ui(:,iiuav),2) * Ri(:,:,iiuav) * e3;

== matlab function sim_pos_dist_obs_tcas/cal x2_hat agent 2 ==
  data: k0 input; k2v input; d_x2_hat_2 output; ell2 input; epv input; Ri input; ui input; dp_hat_vec input; x1_tilt_vec input; G_fun_x1_tilt_2_vec input
function d_x2_hat_2 = fcn(k0, k2v, ell2, epv, Ri, ui, dp_hat_vec, x1_tilt_vec, G_fun_x1_tilt_2_vec)
%%%% 计算状态观测误差
iiuav = 2;
g0 = 9.80663;
e3 = [0;0;1];
d_x2_hat_2 = dp_hat_vec(:,iiuav) + k2v(:) .* ( (x1_tilt_vec(:,iiuav) ./ (epv(:) .^ 2)) + ...
                                                                (k0(:) .^ 2) .* ell2(:) .* G_fun_x1_tilt_2_vec(:,iiuav) ) + ...
                                                                - g0 * e3 + norm(ui(:,iiuav),2) * Ri(:,:,iiuav) * e3;

== matlab function sim_pos_dist_obs_tcas/trans to column2 ==
  data: x input; y output
function y = fcn(x)
y = x(:);

== matlab function sim_pos_dist_obs_tcas/cal x2_hat agent 3 ==
  data: k0 input; k2v input; d_x2_hat_3 output; ell2 input; epv input; Ri input; ui input; dp_hat_vec input; x1_tilt_vec input; G_fun_x1_tilt_2_vec input
function d_x2_hat_3 = fcn(k0, k2v, ell2, epv, Ri, ui, dp_hat_vec, x1_tilt_vec, G_fun_x1_tilt_2_vec)
%%%% 计算状态观测误差
iiuav = 3;
g0 = 9.80663;
e3 = [0;0;1];
d_x2_hat_3 = dp_hat_vec(:,iiuav) + k2v(:) .* ( (x1_tilt_vec(:,iiuav) ./ (epv(:) .^ 2)) + ...
                                                                (k0(:) .^ 2) .* ell2(:) .* G_fun_x1_tilt_2_vec(:,iiuav) ) + ...
                                                                - g0 * e3 + norm(ui(:,iiuav),2) * Ri(:,:,iiuav) * e3;

== matlab function sim_pos_dist_obs_tcas/cal x2_hat agent 4 ==
  data: k0 input; k2v input; d_x2_hat_4 output; ell2 input; epv input; Ri input; ui input; dp_hat_vec input; x1_tilt_vec input; G_fun_x1_tilt_2_vec input
function d_x2_hat_4 = fcn(k0, k2v, ell2, epv, Ri, ui, dp_hat_vec, x1_tilt_vec, G_fun_x1_tilt_2_vec)
%%%% 计算状态观测误差
iiuav = 4;
g0 = 9.80663;
e3 = [0;0;1];
d_x2_hat_4 = dp_hat_vec(:,iiuav) + k2v(:) .* ( (x1_tilt_vec(:,iiuav) ./ (epv(:) .^ 2)) + ...
                                                                (k0(:) .^ 2) .* ell2(:) .* G_fun_x1_tilt_2_vec(:,iiuav) ) + ...
                                                                - g0 * e3 + norm(ui(:,iiuav),2) * Ri(:,:,iiuav) * e3;

== matlab function sim_pos_dist_obs_tcas/cal x2_hat agent 5 ==
  data: k0 input; k2v input; d_x2_hat_5 output; ell2 input; epv input; Ri input; ui input; dp_hat_vec input; x1_tilt_vec input; G_fun_x1_tilt_2_vec input
function d_x2_hat_5 = fcn(k0, k2v, ell2, epv, Ri, ui, dp_hat_vec, x1_tilt_vec, G_fun_x1_tilt_2_vec)
%%%% 计算状态观测误差
iiuav = 5;
g0 = 9.80663;
e3 = [0;0;1];
d_x2_hat_5 = dp_hat_vec(:,iiuav) + k2v(:) .* ( (x1_tilt_vec(:,iiuav) ./ (epv(:) .^ 2)) + ...
                                                                (k0(:) .^ 2) .* ell2(:) .* G_fun_x1_tilt_2_vec(:,iiuav) ) + ...
                                                                - g0 * e3 + norm(ui(:,iiuav),2) * Ri(:,:,iiuav) * e3;

== matlab function sim_pos_dist_obs_tcas/combine x2_hat ==
  data: x2_hat_1 input; x2_hat_2 input; x2_hat_3 input; x2_hat_4 input; x2_hat_5 input; x2_hat_vec output
function x2_hat_vec  = fcn(x2_hat_1, x2_hat_2, x2_hat_3, x2_hat_4, x2_hat_5)
%%%% 合并领导者位置观测器输出结果
x2_hat_vec = [x2_hat_1(:), x2_hat_2(:), x2_hat_3(:), x2_hat_4(:), x2_hat_5(:)];

== matlab function sim_pos_dist_obs_tcas/cal dp_hat agent 1 ==
  data: k0 input; k3v input; dp_hat_1 output; ell3 input; epv input; x1_tilt_vec input; G_fun_x1_tilt_3_vec input
function dp_hat_1 = fcn(k0, k3v, ell3, epv, x1_tilt_vec, G_fun_x1_tilt_3_vec)
%%%% 计算状态观测误差
iiuav = 1;
dp_hat_1 = k3v(:) .* ( (x1_tilt_vec(:,iiuav) ./ (epv(:) .^ 3)) + ...
                    ((k0(:) .^ 3) ./ (ell3(:) .* epv(:))) .* G_fun_x1_tilt_3_vec(:,iiuav) );

== matlab function sim_pos_dist_obs_tcas/trans to column3 ==
  data: x input; y output
function y = fcn(x)
y = x(:);

== matlab function sim_pos_dist_obs_tcas/cal dp_hat agent 2 ==
  data: k0 input; k3v input; dp_hat_2 output; ell3 input; epv input; x1_tilt_vec input; G_fun_x1_tilt_3_vec input
function dp_hat_2 = fcn(k0, k3v, ell3, epv, x1_tilt_vec, G_fun_x1_tilt_3_vec)
%%%% 计算状态观测误差
iiuav = 2;
dp_hat_2 = k3v(:) .* ( (x1_tilt_vec(:,iiuav) ./ (epv(:) .^ 3)) + ...
                    ((k0(:) .^ 3) ./ (ell3(:) .* epv(:))) .* G_fun_x1_tilt_3_vec(:,iiuav) );

== matlab function sim_pos_dist_obs_tcas/cal dp_hat agent 3 ==
  data: k0 input; k3v input; dp_hat_3 output; ell3 input; epv input; x1_tilt_vec input; G_fun_x1_tilt_3_vec input
function dp_hat_3 = fcn(k0, k3v, ell3, epv, x1_tilt_vec, G_fun_x1_tilt_3_vec)
%%%% 计算状态观测误差
iiuav = 3;
dp_hat_3 = k3v(:) .* ( (x1_tilt_vec(:,iiuav) ./ (epv(:) .^ 3)) + ...
                    ((k0(:) .^ 3) ./ (ell3(:) .* epv(:))) .* G_fun_x1_tilt_3_vec(:,iiuav) );

== matlab function sim_pos_dist_obs_tcas/cal dp_hat agent 4 ==
  data: k0 input; k3v input; dp_hat_4 output; ell3 input; epv input; x1_tilt_vec input; G_fun_x1_tilt_3_vec input
function dp_hat_4 = fcn(k0, k3v, ell3, epv, x1_tilt_vec, G_fun_x1_tilt_3_vec)
%%%% 计算状态观测误差
iiuav = 4;
dp_hat_4 = k3v(:) .* ( (x1_tilt_vec(:,iiuav) ./ (epv(:) .^ 3)) + ...
                    ((k0(:) .^ 3) ./ (ell3(:) .* epv(:))) .* G_fun_x1_tilt_3_vec(:,iiuav) );

== matlab function sim_pos_dist_obs_tcas/cal dp_hat agent 5 ==
  data: k0 input; k3v input; dp_hat_5 output; ell3 input; epv input; x1_tilt_vec input; G_fun_x1_tilt_3_vec input
function dp_hat_5 = fcn(k0, k3v, ell3, epv, x1_tilt_vec, G_fun_x1_tilt_3_vec)
%%%% 计算状态观测误差
iiuav = 5;
dp_hat_5 = k3v(:) .* ( (x1_tilt_vec(:,iiuav) ./ (epv(:) .^ 3)) + ...
                    ((k0(:) .^ 3) ./ (ell3(:) .* epv(:))) .* G_fun_x1_tilt_3_vec(:,iiuav) );

== matlab function sim_pos_dist_obs_tcas/trans to column78 ==
  data: x input; y output
function y = fcn(x)
y = x(:);

== matlab function sim_pos_dist_obs_tcas/trans to column79 ==
  data: x input; y output
function y = fcn(x)
y = x(:);

== matlab function sim_pos_dist_obs_tcas/cal abs 5 ==
  data: x input; y output
function y = fcn(x)
y = abs(x(:));

== matlab function sim_pos_dist_obs_tcas/trans to column80 ==
  data: x input; y output
function y = fcn(x)
y = x(:);

== matlab function sim_pos_dist_obs_tcas/combine dp_hat ==
  data: dp_hat_1 input; dp_hat_2 input; dp_hat_3 input; dp_hat_4 input; dp_hat_5 input; dp_hat_vec output
function dp_hat_vec  = fcn(dp_hat_1, dp_hat_2, dp_hat_3, dp_hat_4, dp_hat_5)
%%%% 合并扰动观测值dp_hat
dp_hat_vec = [dp_hat_1(:), dp_hat_2(:), dp_hat_3(:), dp_hat_4(:), dp_hat_5(:)];

== matlab function sim_pos_dist_obs_tcas/cal abs 31 ==
  data: x input; y output
function y = fcn(x)
y = abs(x(:));

== matlab function sim_pos_dist_obs_tcas/cal abs 32 ==
  data: x input; y output
function y = fcn(x)
y = abs(x(:));

== matlab function sim_pos_dist_obs_tcas/cal theta_phi agent 1 ==
  data: alfa_theta input; phi_squ_1_1 input; theta_phi_1_1 output; phi_squ_2_1 input; phi_vec input; theta_phi_2_1 output
function [theta_phi_1_1, theta_phi_2_1] = fcn(alfa_theta, phi_squ_1_1, phi_squ_2_1, phi_vec)
%%%% 计算平滑递增函数
iiuav = 1;
theta_phi_1_1 = phi_squ_1_1(:) .* ( -1 + 2 ./ ( 1 + exp( -alfa_theta .* phi_vec(:,iiuav) ) ) );
theta_phi_2_1 = phi_squ_2_1(:) .* ( -1 + 2 ./ ( 1 + exp( -alfa_theta .* phi_vec(:,iiuav) ) ) );

== matlab function sim_pos_dist_obs_tcas/choose ksi_est_err 31 ==
  data: x input; y output
function y = fcn(x)
iiuav = 1;
y = x(:,iiuav);

== matlab function sim_pos_dist_obs_tcas/choose ksi_est_err 32 ==
  data: x input; y output
function y = fcn(x)
iiuav = 1;
y = x(:,iiuav);

== matlab function sim_pos_dist_obs_tcas/trans to column30 ==
  data: x input; y output
function y = fcn(x)
y = x(:);

== matlab function sim_pos_dist_obs_tcas/trans to column31 ==
  data: x input; y output
function y = fcn(x)
y = x(:);

== matlab function sim_pos_dist_obs_tcas/cal G_fun_x1_tilt agent 1 ==
  data: err_1_x1_tilt_vec input; err_2_x1_tilt_vec input; G_fun_x1_tilt_1_1 output; err_3_x1_tilt_vec input; err_x1_alfa_squ_1_1 input; G_fun_x1_tilt_2_1 output; err_x1_alfa_squ_2_1 input; err_x1_alfa_squ_3_1 input; err_x1_alfa_squ_4_1 input; err_x1_alfa_squ_5_1 input; err_x1_alfa_squ_6_1 input; G_fun_x1_tilt_3_1 output
function [G_fun_x1_tilt_1_1, G_fun_x1_tilt_2_1, G_fun_x1_tilt_3_1] = fcn(err_1_x1_tilt_vec, err_2_x1_tilt_vec, err_3_x1_tilt_vec, ...
                                                                                                                                err_x1_alfa_squ_1_1, err_x1_alfa_squ_2_1, err_x1_alfa_squ_3_1, ...
                                                                                                                                err_x1_alfa_squ_4_1, err_x1_alfa_squ_5_1, err_x1_alfa_squ_6_1)
%%%% 计算平滑递增函数
iiuav = 1;
G_fun_x1_tilt_1_1 = tanh(err_x1_alfa_squ_2_1(:)) .* err_x1_alfa_squ_1_1(:) .* sign(err_1_x1_tilt_vec(:,iiuav));
G_fun_x1_tilt_2_1 = tanh(err_x1_alfa_squ_4_1(:)) .* err_x1_alfa_squ_3_1(:) .* sign(err_2_x1_tilt_vec(:,iiuav));
G_fun_x1_tilt_3_1 = tanh(err_x1_alfa_squ_6_1(:)) .* err_x1_alfa_squ_5_1(:) .* sign(err_3_x1_tilt_vec(:,iiuav));

== matlab function sim_pos_dist_obs_tcas/cal abs 33 ==
  data: x input; y output
function y = fcn(x)
y = abs(x(:));

== matlab function sim_pos_dist_obs_tcas/cal abs 34 ==
  data: x input; y output
function y = fcn(x)
y = abs(x(:));

== matlab function sim_pos_dist_obs_tcas/cal theta_phi agent 2 ==
  data: alfa_theta input; phi_squ_1_2 input; theta_phi_1_2 output; phi_squ_2_2 input; phi_vec input; theta_phi_2_2 output
function [theta_phi_1_2, theta_phi_2_2] = fcn(alfa_theta, phi_squ_1_2, phi_squ_2_2, phi_vec)
%%%% 计算平滑递增函数
iiuav = 2;
theta_phi_1_2 = phi_squ_1_2(:) .* ( -1 + 2 ./ ( 1 + exp( -alfa_theta .* phi_vec(:,iiuav) ) ) );
theta_phi_2_2 = phi_squ_2_2(:) .* ( -1 + 2 ./ ( 1 + exp( -alfa_theta .* phi_vec(:,iiuav) ) ) );

== matlab function sim_pos_dist_obs_tcas/choose ksi_est_err 33 ==
  data: x input; y output
function y = fcn(x)
iiuav = 2;
y = x(:,iiuav);

== matlab function sim_pos_dist_obs_tcas/choose ksi_est_err 34 ==
  data: x input; y output
function y = fcn(x)
iiuav = 2;
y = x(:,iiuav);

== matlab function sim_pos_dist_obs_tcas/trans to column32 ==
  data: x input; y output
function y = fcn(x)
y = x(:);

== matlab function sim_pos_dist_obs_tcas/trans to column33 ==
  data: x input; y output
function y = fcn(x)
y = x(:);

== matlab function sim_pos_dist_obs_tcas/cal abs 35 ==
  data: x input; y output
function y = fcn(x)
y = abs(x(:));

== matlab function sim_pos_dist_obs_tcas/cal abs 36 ==
  data: x input; y output
function y = fcn(x)
y = abs(x(:));

== matlab function sim_pos_dist_obs_tcas/cal theta_phi agent 3 ==
  data: alfa_theta input; phi_squ_1_3 input; theta_phi_1_3 output; phi_squ_2_3 input; phi_vec input; theta_phi_2_3 output
function [theta_phi_1_3, theta_phi_2_3] = fcn(alfa_theta, phi_squ_1_3, phi_squ_2_3, phi_vec)
%%%% 计算平滑递增函数
iiuav = 3;
theta_phi_1_3 = phi_squ_1_3(:) .* ( -1 + 2 ./ ( 1 + exp( -alfa_theta .* phi_vec(:,iiuav) ) ) );
theta_phi_2_3 = phi_squ_2_3(:) .* ( -1 + 2 ./ ( 1 + exp( -alfa_theta .* phi_vec(:,iiuav) ) ) );

== matlab function sim_pos_dist_obs_tcas/choose ksi_est_err 35 ==
  data: x input; y output
function y = fcn(x)
iiuav = 3;
y = x(:,iiuav);

== matlab function sim_pos_dist_obs_tcas/choose ksi_est_err 36 ==
  data: x input; y output
function y = fcn(x)
iiuav = 3;
y = x(:,iiuav);

== matlab function sim_pos_dist_obs_tcas/trans to column34 ==
  data: x input; y output
function y = fcn(x)
y = x(:);

== matlab function sim_pos_dist_obs_tcas/trans to column36 ==
  data: x input; y output
function y = fcn(x)
y = x(:);

== matlab function sim_pos_dist_obs_tcas/cal abs 37 ==
  data: x input; y output
function y = fcn(x)
y = abs(x(:));

== matlab function sim_pos_dist_obs_tcas/cal abs 38 ==
  data: x input; y output
function y = fcn(x)
y = abs(x(:));

== matlab function sim_pos_dist_obs_tcas/cal theta_phi agent 4 ==
  data: alfa_theta input; phi_squ_1_4 input; theta_phi_1_4 output; phi_squ_2_4 input; phi_vec input; theta_phi_2_4 output
function [theta_phi_1_4, theta_phi_2_4] = fcn(alfa_theta, phi_squ_1_4, phi_squ_2_4, phi_vec)
%%%% 计算平滑递增函数
iiuav = 4;
theta_phi_1_4 = phi_squ_1_4(:) .* ( -1 + 2 ./ ( 1 + exp( -alfa_theta .* phi_vec(:,iiuav) ) ) );
theta_phi_2_4 = phi_squ_2_4(:) .* ( -1 + 2 ./ ( 1 + exp( -alfa_theta .* phi_vec(:,iiuav) ) ) );

== matlab function sim_pos_dist_obs_tcas/choose ksi_est_err 37 ==
  data: x input; y output
function y = fcn(x)
iiuav = 4;
y = x(:,iiuav);

== matlab function sim_pos_dist_obs_tcas/choose ksi_est_err 38 ==
  data: x input; y output
function y = fcn(x)
iiuav = 4;
y = x(:,iiuav);

== matlab function sim_pos_dist_obs_tcas/trans to column37 ==
  data: x input; y output
function y = fcn(x)
y = x(:);

== matlab function sim_pos_dist_obs_tcas/trans to column38 ==
  data: x input; y output
function y = fcn(x)
y = x(:);

== matlab function sim_pos_dist_obs_tcas/cal abs 39 ==
  data: x input; y output
function y = fcn(x)
y = abs(x(:));

== matlab function sim_pos_dist_obs_tcas/cal abs 40 ==
  data: x input; y output
function y = fcn(x)
y = abs(x(:));
